simulink model "RCcircuit"  (R2020a)
settings: Solver=ode3  StartTime=0.0  StopTime=5  FixedStep=0.001  RelTol=1e-3
model workspace (MAT data in the model file):
  C = 0.0001
  R = 1500
settings Model: OrderedModelArguments=off  Creator=shaun  LastModifiedBy=shaun

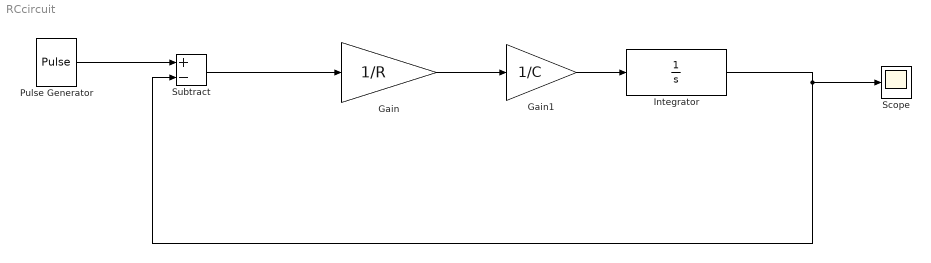
== system RCcircuit ==
  Gain : Gain  Gain=1/R
  Gain1 : Gain  Gain=1/C
  Integrator : Integrator
  Pulse Generator : DiscretePulseGenerator  PulseType=Time based  Amplitude=5  PulseWidth=50
  Scope : Scope
  Subtract : Sum  Inputs=+-
  wires:
  Pulse Generator/1 -> Subtract/1
  Subtract/1 -> Gain/1
  Gain/1 -> Gain1/1
  Gain1/1 -> Integrator/1
  Integrator/1 -> Subtract/2, Scope/1
